simulink model "Model"  (R2024b)
settings: Solver=ode45  StartTime=0.0  StopTime=10.0  RelTol=1e-3
InitFcn:
  | Main
values from neighbouring files (symbols this model uses):
  A = P.A    [Main.m]
  Ao = Ad - L*Cd    [Main.m]
  B = P.B    [Main.m]
  Bo = [Bd, L]    [Main.m]
  C = P.C    [Main.m]
  Co = eye(2)    [Main.m]
  D = P.D    [Main.m]
  Do = zeros(2)    [Main.m]
  K = place(Ad, Bd, CtrlPolesZ)    [Main.m]
  Nr = Nu + K*Nx    [Main.m]
  Ts = RiseTime / 30    (= 0.00833333333333)    [Main.m]
settings Model: Creator=Banaan  LastModifiedBy=Banaan

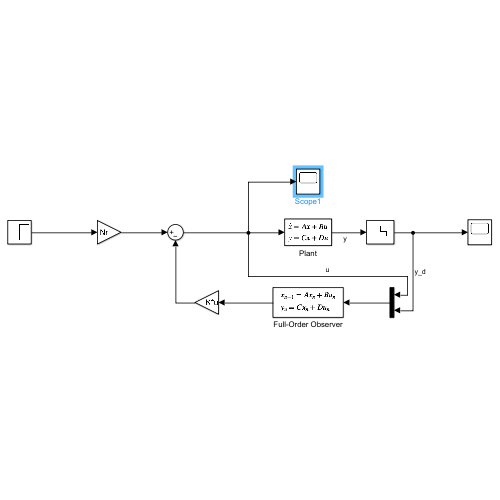
[thumbnail: Simulink's stored preview of the top-level diagram]
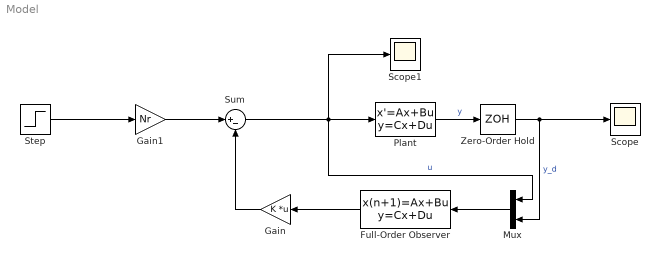
== system Model ==
  Full-Order Observer : DiscreteStateSpace  A=Ao  B=Bo  C=Co  D=Do  SampleTime=Ts
  Gain : Gain  Gain=K  Multiplication=Matrix(K*u)
  Gain1 : Gain  Gain=Nr
  Mux : Mux  Inputs=2
  Plant : StateSpace  A=A  B=B  C=C  D=D  InitialCondition=0
  Scope : Scope
  Scope1 : Scope
  Step : Step  SampleTime=0
  Sum : Sum  Inputs=|+-
  Zero-Order Hold : ZeroOrderHold  SampleTime=Ts
  wires:
  Plant/1 -> Zero-Order Hold/1  "y"
  Full-Order Observer/1 -> Gain/1
  Gain/1 -> Sum/2
  Sum/1 -> Plant/1, Mux/1, Scope1/1  "u"
  Gain1/1 -> Sum/1
  Step/1 -> Gain1/1
  Mux/1 -> Full-Order Observer/1
  Zero-Order Hold/1 -> Mux/2, Scope/1  "y_d"
